simulink model "main_vehicle_v2"  (R2024b)
settings: Solver=FixedStepAuto  StartTime=0.0  StopTime=5  FixedStep=Ts  MaxStep=0.001  RelTol=1e-3
values from neighbouring files (symbols this model uses):
  Frr = Crr*m*g    (= 51.993)    [main_data_vehicle.m]    (also in xopt_launch.mat)
  lf = L*fr    (= 0.7905)    [main_data_vehicle.m]    (also in xopt_launch.mat)
  Re = 0.235    [main_data_vehicle.m]    (also in xopt_launch.mat)
  t_vec = (0:dt:simTime)'    [buildControlProfile.m]    (also in buildControlProfile2.m; optimal_launch_pedal_goodyear.mat = [0 0.001 0.002 0.003 0.004 0.005 0.006 0.007 0.008 0.009 0.0; optimal_launch_pedal_refined.mat = [0 0.001 0.002 0.003 0.004 0.005 0.006 0.007 0.008 0.009 0.0; optimal_launch_pedal_result.mat = [0 0.001 0.002 0.003 0.004 0.005 0.006 0.007 0.008 0.009 0.0)
  TirePressure = 65e3    (= 65000)    [main_data_vehicle.m]    (also in xopt_launch.mat)
  Ts = 0.001    [main_data_vehicle.m]    (also in xopt_launch.mat)
  u_vec = min(max(u_vec, uMin), uMax)    [buildControlProfile.m]    (also in buildControlProfile2.m; optimal_launch_pedal_goodyear.mat = [0.4076171875 0.409837690443 0.412058165147 0.414278583859 0; optimal_launch_pedal_refined.mat = [0.90859375 0.907017815717 0.905446650732 0.903880250909 0.9; optimal_launch_pedal_result.mat = [0.2 0.202202584529 0.204404077869 0.206604464652 0.20880372)
  v0 = 0    [main_data_vehicle.m]    (also in xopt_launch.mat)
undefined symbols (not defined in the file or in its folder): Sim3dSensor
libraries: simulink x3, sim3dlib x3, sim3dautolib x1, dspvision x1
settings Model: Creator=marti  LastModifiedBy=marti

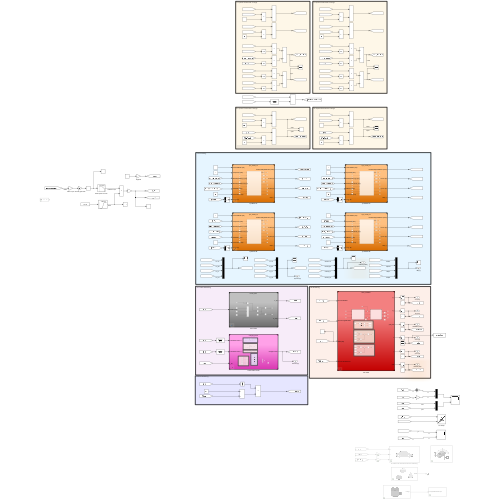
[thumbnail: Simulink's stored preview of the top-level diagram]
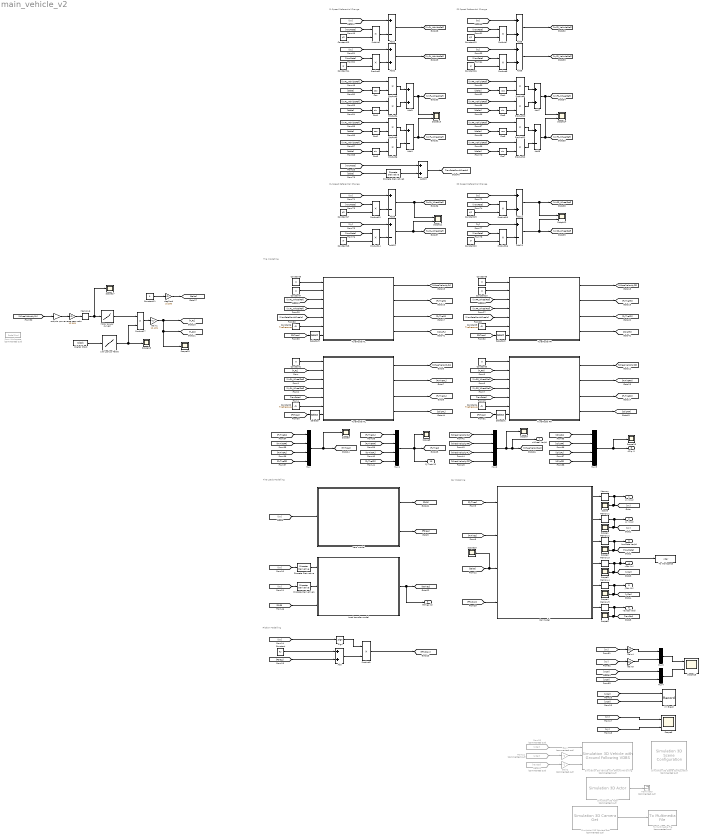
== system main_vehicle_v2 ==
  note: FL Speed Referential Change
  note: Car Modelling
  note: Friction Modelling
  note: Tire Loads Modelling
  note: Tire modelling
  note: FR Speed Referential Change
  note: RL Speed Referential Change
  note: RR Speed Referential Change
  1-D Lookup Table : Lookup_n-D  NumberOfTableDimensions=1  BreakpointsForDimension1=t_vec  Table=u_vec  InternalRulePriority=Speed  RndMeth=Simplest
  Add{,2..3,5..7,12..13} (8 alike) : Sum
  Add{1,4,8..11} (6 alike) : Sum  Inputs=+-
  Aero model : ModelReference  ModelNameDialog=forces_aero.slx  SimulationMode=Normal  ModelReferenceVersion=1.8
  Car model : ModelReference  ModelNameDialog=state_variables.slx  SimulationMode=Normal  ModelReferenceVersion=1.15
  Constant : Constant  Value=Frr
  Constant{1,3,5,7..8,10..11} (7 alike) : Constant  Value=0
  Constant{13,15,17,19} (4 alike) : Constant  Value=t/2
  Constant{14,16,18,20} (4 alike) : Constant  Value=lf
  Constant{2,4,6,9} (4 alike) : Constant  Value=TirePressure
  Cos{,2,4,6} (4 alike) : Trigonometry  Operator=cos
  Cos{1,3,5,7} (4 alike) : Trigonometry
  Digital Clock : DigitalClock  SampleTime=Ts
  Discrete Derivative : simulink/Discrete/Discrete Derivative  gainval=1.0  ICPrevScaledInput=0.0  OutMin=[]  OutMax=[]  OutDataType=fixdt(1, 16)  OutScaling=2^-10  DoSatur=off
  Discrete Derivative1 : simulink/Discrete/Discrete Derivative  gainval=1.0  ICPrevScaledInput=0.0  OutMin=[]  OutMax=[]  OutDataType=fixdt(1, 16)  OutScaling=2^-10  DoSatur=off
  Discrete Derivative2 : simulink/Discrete/Discrete Derivative  gainval=1.0  ICPrevScaledInput=0.0  OutMin=[]  OutMax=[]  OutDataType=fixdt(1, 16)  OutScaling=2^-10  DoSatur=off
  From Workspace : FromWorkspace  Commented=on  VariableName=PedalCmd
  From20 : From  Commented=on  GotoTag=xCar
  From21 : From  Commented=on  GotoTag=yCar
  From22 : From  Commented=on  GotoTag=YawCar
  Gain : Gain  Commented=on  Gain=-1
  Gain1 : Gain  Gain=12.481
  Gain2 : Gain  Commented=on  Gain=-1
  Gain4 : Gain  Gain=3.6
  Gain5 : Gain  Gain=3.6
  Load transfer model : ModelReference  ModelNameDialog=charges_pneus.slx  SimulationMode=Normal  ModelReferenceVersion=1.26
  Memory : Memory  InitialCondition=v0
  Memory{1..5} (5 alike) : Memory
  Memory6 : Memory  InitialCondition=v0/Re
  Motor power curve2 : Lookup_n-D  NumberOfTableDimensions=1  BreakpointsForDimension1=[0 11500 20000 20001]  Table=[32 32 18 0]  ExtrapMethod=Clip  UseLastTableValue=on  InternalRulePriority=Speed  RndMeth=Simplest
  Mux{,1..2,5} (4 alike) : Mux
  Mux3 : Mux  Inputs=2
  Mux4 : Mux  Inputs=2
  Product{,1..17} (18 alike) : Product
  Scope{,1..5,7..10,16..19} (14 alike) : Scope
  Scope{6,11..15} (6 alike) : Scope  NumInputPorts=2
  Selector : Selector  InputPortWidth=4  IndexOptions=Index vector (dialog)  Indices=1  OutputSizes=1
  Selector1 : Selector  InputPortWidth=4  IndexOptions=Index vector (dialog)  Indices=2  OutputSizes=1
  Selector2 : Selector  InputPortWidth=4  IndexOptions=Index vector (dialog)  Indices=4  OutputSizes=1
  Selector3 : Selector  InputPortWidth=4  IndexOptions=Index vector (dialog)  Indices=3  OutputSizes=1
  Sign : Signum
  Simulation 3D Actor : sim3dlib/Simulation 3D Actor  Commented=on  ActorName=Sim3dActor5  ParentName=Scene Origin  Operation=Create at setup  InitScriptText=skidpadConePlacement  SampleTime=.03  Translation=single([0 0 0])  Rotation=single([0 0 0])  Scale=single([1 1 1])  aMode=5  ActorTag=Sim3dActor5  ActorType=Sim3dActor  ID=5
      settings: LibrarySourceBlock=sl3dlib/Simulation 3D/Simulation 3D Actor
  Simulation 3D Camera Get : sim3dlib/Simulation 3D Camera Get  Priority=1  Commented=on  sensorTag=Sim3dSensor�  sensorId=2  sensorName=Sim3dSensor�  vehTagList={'Scene Origin';'Sim3dActor1';'Sim3dActor2';'Sim3dActor3';'Sim3dActor4';'Sim3dActor5';'SimulinkVehicle1'}  vehTag=SimulinkVehicle1  mountLoc=Origin  offsetFlag=on  tmountOffset=[-8, 0, 1]  rmountOffset=[0, 0, 0]  HorizontalResolution=1280  VerticalResolution=720  HorizontalFOV=60  SampleTime=0.03  mountPoint=[-8 0 1]  mountOrientation=[0 0 0]  aMode=5  ID=2
      settings: LibrarySourceBlock=sl3dlib/Simulation 3D/Utilities/Simulation 3D Camera Get
  Simulation 3D Scene Configuration : sim3dlib/Simulation 3D Scene Configuration  Priority=0  Commented=on  ProjectFormat=Default Scenes  SceneDesc=Straight road  ProjectName=C:\Program Files\MATLAB\R2024b\toolbox\shared\sim3d_projects\automotive_project_windows\UE\WindowsNoEditor\VehicleSimulation.exe  ScenePath=/Game/Maps/HwStrght  EnableOpenDRIVE=off  vehTagList={'Custom';'Scene Origin';'Sim3dActor1';'Sim3dActor2';'Sim3dActor3';'Sim3dActor4';'Sim3dActor5';'SimulinkVehicle1'}  vehTag=SimulinkVehicle1  FreeCameraInitialTranslation=[0, 0, 0]  FreeCameraDefaultInitialTranslation=[-6, 0, 2]  FreeCameraInitialRotation=[0, 0, 0]  FreeCameraDefaultInitialRotation=[0, -15, 0]  OpVisEn=off  Ts=.03  EnableWindow=on  EnableRemoteAccess=off  EnableWeather=off  SunAzimuth=90  SunAltitude=40.0  EnableGeospatialSun=off  Latitude=0  Longitude=0  Date=2023-01-01  Time=10:30:00  GeoTimeZone=-5.0  SunDaylightSaving=off  wind=1  clouds=10  EnableVolumetricClouds=off  CloudCoverage=0  CloudAltitude=6  fog=0  rain=0  RaindropsEffect=off  SnowDensity=0  EnableGeospatial=off  UseTrueOrigin=off  OriginHeight=200  OriginLatitude=40.744652  OriginLongitude=-73.988864  MapStyle=Aerial  AdditionalAssetIDs=[]  UseAdvancedSunSky=off  SolarTime=11  TimeZone=-5  Day=21  Month=9  Year=2022  UseDaylightSavingTime=on  DSTStartDay=10  DSTStartMonth=3  DSTEndDay=3  DSTEndMonth=11  DSTSwitchHour=2  sensorTag=MainCamera1  sensorId=1  sensorName=MainCamera1  mountLoc=Origin  offsetFlag=off  tmountOffset=[0, 0, 0]  rmountOffset=[0, 0, 0]  HorizontalResolution=1280  VerticalResolution=720  HorizontalFOV=60  mountPoint=[0 0 0]  mountOrientation=[0 0 0]  aMode=2  ID=1  GeoTrigger=Inactive
      settings: LibrarySourceBlock=vehdynlibsim3dcore/Simulation 3D Scene Configuration
  Simulation 3D Vehicle with Ground Following : sim3dautolib/Simulation 3D Vehicle with Ground Following VDBS  Priority=-1  Commented=on  PassVehMesh=Formula student vehicle  MeshPath=/MathWorksAutomotiveContent/Vehicles/Muscle/Meshes/SK_MuscleCar.SK_MuscleCar  TrackWidth=1.9  WheelBase=3  WheelRadius=0.35  VehColor=Silver  InitialPos=[0, 0, 0]  InitialRot=[0, 0, 0]  ActorName=SimulinkVehicle1  VehLightsControl=off  HeadlightColor=[ 1, 1, 1 ]  HighBeamIntensity=100000  LowBeamIntensity=60000  HighBeamConeAngle=1.22  LowBeamConeAngle=1.22  LeftHeadlightOrientation=[ 0, 0 ]  RightHeadlightOrientation=[ 0, 0 ]  BrakelightIntensity=200  ReverselightIntensity=500  SignallightIntensity=500  SignallightPeriod=1  SignalPulseWidth=50  SampleTime=-1  ActorType=SimulinkVehicle  ID=1  aMode=2  ActorTag=SimulinkVehicle1  CoordinateScheme=SAE
      settings: LibrarySourceBlock=vehdynlibsim3d/Simulation 3D Vehicle with Ground Following
  Terminator : Terminator  Commented=on
  To Multimedia File : dspvision/To Multimedia File  Commented=on  outputFilename=C:\Users\marti\Documents\EPSA\Travaux torque structure\SKIDPAD.mp4  streamSelection=Video only  videoCompressor=None (uncompressed)  audioCompressor=None (uncompressed)  imagePorts=One multidimensional signal  fileType=MPEG4  audioDatatype=Determine from input data type  fourcc=RGB  audioBitRate=128  audioQuality=75  videoQuality=75  mj2000CompFactor=10
      settings: LibrarySourceBlock=visionsinks/To Multimedia File
  To Workspace : ToWorkspace  VariableName=xCar  SaveFormat=Timeseries  SampleTime=Ts
  TyreModel FL : ModelReference  ModelNameDialog=tyre_model_v3.slx  SimulationMode=Normal  ModelReferenceVersion=1.26
  TyreModel FR : ModelReference  ModelNameDialog=tyre_model_v3.slx  SimulationMode=Normal  ModelReferenceVersion=1.26
  TyreModel RL : ModelReference  ModelNameDialog=tyre_model_v3.slx  SimulationMode=Normal  ModelReferenceVersion=1.26
  TyreModel RR : ModelReference  ModelNameDialog=tyre_model_v3.slx  SimulationMode=Normal  ModelReferenceVersion=1.26
  XY Graph : Record  FileSettingsInternal="{\"entries\":[{\"content\":{\"excelSettings\":{\"content\":{},\"type\":\"Streamout.ExcelSettings\"}},\"type\":\"Streamout.FileSettingStorage\",\"uuid\":\"\"}],\"packageUris\":[\"http:\\/\\/schema.mathworks.com\\/mf0\\/streamout_blocks\\/R2020a\"],\"version\":\"1.0\"}"  Layout=[1 1]  SignalsInternal="{\"entries\":[{\"content\":{\"signals\":[{\"content\":{\"blockPath\":[],\"dimensions\":[1],\"domain\":\"\",\"lineColor\":\"#0072bd\",\"lineWidth\":2,\"plots\":[ 1 ],\"port\":1,\"sid\":[\"\"],\"signalID\":1,\"signalName\":\"From16\"},\"type\":\"RecordBlkView.Signal\",\"uuid\":\"\"},{\"content\":{\"blockPath\":[],\"dimensions\":[1],\"domain\":\"\",\"lineColor\":\"#d95319\",\"lineWidth\":2,\"plots\":[ 1 ],\"port\":2,\"sid\":[\"\"],\"signalID\":2,\"signalName\":\"From15\"},\"type\":\"RecordBlkView.Signal\",\"uuid\":\"\"}]},\"type\":\"RecordBlkView.InputSignals\",\"uuid\":\"\"}],\"packageUris\":[\"http:\\/\\/schema.mathworks.com\\/mf0\\/streamout_blocks\\/R2020a\"],\"version\":\"1.0\"}"  VisualizationBindings="{\"xyplotplugin\":{\"info\":[{\"series\":[{\"bindingParametersList\":[{\"parameter\":\"X-Axis\",\"signalID\":1,\"signalName\":\"From16\"},{\"parameter\":\"Y-Axis\",\"signalID\":2,\"signalName\":\"From15\"}],\"seriesID\":0}],\"subplotID\":1}]}}"  CompatibilityTag=XY
  deg2rad : Gain  Gain=pi/180
  rad/s to rpm : Gain  Gain=30/pi
  reverse gear ratio : Gain  Gain=12.481
  Vx (m/s) : Outport
  Vy (m/s) : Outport  Port=2
  YawRate (rad/s) : Outport  Port=3
  xCar (m) : Outport  Port=4
  yCar (m) : Outport  Port=5
  YawCar (rad) : Outport  Port=6
  nWheel (rad/s) : Outport  Port=7
  rSlip (-) : Outport  Port=8
  FzTires (N) : Outport  Port=9
  FyTires (N) : Outport  Port=10
  wires:
  Car model/1 -> Memory/1
  Car model/2 -> Memory1/1
  Car model/3 -> Memory2/1
  Car model/4 -> Memory3/1
  Car model/5 -> Memory4/1
  Car model/6 -> Memory5/1
  [Vx] -> Aero model/1
  Memory/1 -> Vx (m/s)/1, Scope/1, [Vx]
  Memory1/1 -> Vy (m/s)/1, Scope1/1, [Vy]
  Memory2/1 -> YawRate (rad/s)/1, [YawRate], Scope2/1
  Memory3/1 -> To Workspace/1, xCar (m)/1, Scope3/1, [xCar]
  Memory4/1 -> yCar (m)/1, [yCar], Scope4/1
  Memory5/1 -> YawCar (rad)/1, Scope5/1, [YawCar]
  [Vx] -> Discrete Derivative/1
  Discrete Derivative/1 -> Load transfer model/1
  [Vy] -> Discrete Derivative1/1
  Discrete Derivative1/1 -> Load transfer model/2
  [FxTires] -> Car model/2
  [FyTires] -> Car model/1
  [delta] -> Scope10/1, Car model/3
  Aero model/2 -> [FDrag]
  [FDrag] -> Add/2
  Constant/1 -> Add/1
  [FFriction] -> Car model/4
  Add/1 -> Product1/2
  Load transfer model/1 -> FzTires (N)/1, [FzTires]
  [Vx] -> Sign/1
  Sign/1 -> Product1/1
  [yCar] -> XY Graph/2
  [xCar] -> XY Graph/1
  [Vx] -> Scope6/1  "v_x"
  [Vy] -> Scope6/2  "v_y"
  From20/1 -> Simulation 3D Vehicle with Ground Following/1
  From21/1 -> Gain/1
  From22/1 -> Gain2/1
  Gain/1 -> Simulation 3D Vehicle with Ground Following/2
  Gain2/1 -> Simulation 3D Vehicle with Ground Following/3
  Simulation 3D Actor/1 -> Terminator/1
  Simulation 3D Camera Get/1 -> To Multimedia File/1
  Constant1/1 -> TyreModel RL/1
  [T_RL] -> TyreModel RL/2
  [VxRL_WheelRef] -> TyreModel RL/3
  [VyRL_WheelRef] -> TyreModel RL/4
  [YawRate] -> TyreModel RL/5
  Constant2/1 -> TyreModel RL/6
  TyreModel RL/1 -> [WheelVelocityRL]
  TyreModel RL/2 -> [FxTireRL]
  TyreModel RL/3 -> [FyTireRL]
  TyreModel RR/3 -> [FyTireRR]
  TyreModel RR/2 -> [FxTireRR]
  TyreModel RR/1 -> [WheelVelocityRR]
  Constant4/1 -> TyreModel RR/6
  [YawRate] -> TyreModel RR/5
  [VyRR_WheelRef] -> TyreModel RR/4
  [VxRR_WheelRef] -> TyreModel RR/3
  [T_RR] -> TyreModel RR/2
  Constant3/1 -> TyreModel RR/1
  TyreModel FL/3 -> [FyTireFL]
  TyreModel FL/2 -> [FxTireFL]
  TyreModel FL/1 -> [WheelVelocityFL]
  Constant6/1 -> TyreModel FL/6
  [YawRateFrontWheels] -> TyreModel FL/5
  [VyFL_WheelRef] -> TyreModel FL/4
  [VxFL_WheelRef] -> TyreModel FL/3
  Constant7/1 -> TyreModel FL/2
  Constant5/1 -> TyreModel FL/1
  Constant8/1 -> TyreModel FR/1
  Constant10/1 -> TyreModel FR/2
  [VxFR_WheelRef] -> TyreModel FR/3
  [VyFR_WheelRef] -> TyreModel FR/4
  [YawRateFrontWheels] -> TyreModel FR/5
  Constant9/1 -> TyreModel FR/6
  TyreModel FR/1 -> [WheelVelocityFR]
  TyreModel FR/2 -> [FxTireFR]
  TyreModel FR/3 -> [FyTireFR]
  Aero model/1 -> [FLift]
  Product1/1 -> [FFriction]
  [FzTires] -> Selector/1
  Selector/1 -> TyreModel RL/7
  [FzTires] -> Selector1/1
  Selector1/1 -> TyreModel RR/7
  [FzTires] -> Selector2/1
  Selector2/1 -> TyreModel FR/7
  [FzTires] -> Selector3/1
  Selector3/1 -> TyreModel FL/7
  [FxTireRL] -> Mux/1  "Fx_RL"
  [FxTireRR] -> Mux/2  "Fx_RR"
  [FxTireFL] -> Mux/3  "Fx_FL"
  [FxTireFR] -> Mux/4  "Fx_FR"
  Mux/1 -> Scope9/1, [FxTires]
  Mux1/1 -> FyTires (N)/1, Scope8/1, [FyTires]
  [FyTireFR] -> Mux1/4  "Fy_FR"
  [FyTireFL] -> Mux1/3  "Fy_FL"
  [FyTireRR] -> Mux1/2  "Fy_RR"
  [FyTireRL] -> Mux1/1  "Fy_RL"
  Mux2/1 -> Scope7/1, nWheel (rad/s)/1, [WheelVelocities]
  [WheelVelocityRL] -> Mux2/1  "nWheel_RL"
  [WheelVelocityRR] -> Mux2/2  "nWheel_RR"
  [WheelVelocityFL] -> Mux2/3  "nWheel_FL"
  [WheelVelocityFR] -> Mux2/4  "nWheel_FR"
  [FLift] -> Load transfer model/3
  [Vx] -> Add1/1
  Product/1 -> Add1/2
  [YawRate] -> Product/1
  Constant13/1 -> Product/2
  Add1/1 -> [VxFL_VehicleRef]
  Add2/1 -> [VyFL_VehicleRef]
  Constant14/1 -> Product2/2
  [YawRate] -> Product2/1
  Product2/1 -> Add2/2
  [Vy] -> Add2/1
  [delta] -> Cos/1
  Cos/1 -> Product3/2
  [VxFL_VehicleRef] -> Product3/1
  [VyFL_VehicleRef] -> Product4/1
  Cos1/1 -> Product4/2
  [delta] -> Cos1/1
  Product3/1 -> Add3/1
  Product4/1 -> Add3/2
  Add3/1 -> Scope13/1, [VxFL_WheelRef]  "VxFL"
  Add4/1 -> Scope13/2, [VyFL_WheelRef]  "VyFL"
  Product6/1 -> Add4/2
  Product5/1 -> Add4/1
  [delta] -> Cos3/1
  Cos3/1 -> Product6/2
  [VxFL_VehicleRef] -> Product6/1
  [VyFL_VehicleRef] -> Product5/1
  Cos2/1 -> Product5/2
  [delta] -> Cos2/1
  [delta] -> Cos6/1
  Cos6/1 -> Product11/2
  [VyFR_VehicleRef] -> Product11/1
  [VxFR_VehicleRef] -> Product12/1
  Cos7/1 -> Product12/2
  [delta] -> Cos7/1
  Product11/1 -> Add8/1
  Product12/1 -> Add8/2
  Add8/1 -> Scope14/2, [VyFR_WheelRef]  "VyFR"
  Product10/1 -> Add7/2
  Product9/1 -> Add7/1
  [delta] -> Cos5/1
  Cos5/1 -> Product10/2
  [VyFR_VehicleRef] -> Product10/1
  [VxFR_VehicleRef] -> Product9/1
  Cos4/1 -> Product9/2
  [delta] -> Cos4/1
  [Vy] -> Add6/1
  Product8/1 -> Add6/2
  [YawRate] -> Product8/1
  Constant16/1 -> Product8/2
  Add6/1 -> [VyFR_VehicleRef]
  Add5/1 -> [VxFR_VehicleRef]
  Constant15/1 -> Product7/2
  [YawRate] -> Product7/1
  Product7/1 -> Add5/2
  [Vx] -> Add5/1
  [Vy] -> Add10/1
  Product14/1 -> Add10/2
  [YawRate] -> Product14/1
  Constant18/1 -> Product14/2
  Add10/1 -> Scope11/2, [VyRL_WheelRef]  "VyRL"
  Add9/1 -> Scope11/1, [VxRL_WheelRef]  "VxRL"
  Constant17/1 -> Product13/2
  [YawRate] -> Product13/1
  Product13/1 -> Add9/2
  [Vx] -> Add9/1
  [Vx] -> Add12/1
  Product15/1 -> Add12/2
  [YawRate] -> Product15/1
  Constant19/1 -> Product15/2
  Add12/1 -> Scope12/1, [VxRR_WheelRef]  "VxRR"
  Add11/1 -> Scope12/2, [VyRR_WheelRef]  "VyRR"
  Constant20/1 -> Product16/2
  [YawRate] -> Product16/1
  Product16/1 -> Add11/2
  [Vy] -> Add11/1
  Discrete Derivative2/1 -> Add13/2
  [YawRate] -> Add13/1
  Add13/1 -> [YawRateFrontWheels]
  [delta] -> Discrete Derivative2/1
  Add7/1 -> Scope14/1, [VxFR_WheelRef]  "VxFR"
  Product17/1 -> Gain1/1
  Constant11/1 -> deg2rad/1
  Mux5/1 -> Scope16/1, rSlip (-)/1
  Gain5/1 -> Mux3/2  "v_y"
  Gain4/1 -> Mux3/1  "v_x"
  [Vy] -> Gain5/1  "v_y"
  [Vx] -> Gain4/1  "v_x"
  Mux3/1 -> Scope15/1
  [xCar] -> Mux4/1  "xCar"
  [yCar] -> Mux4/2  "yCar"
  Mux4/1 -> Scope15/2
  deg2rad/1 -> [delta]
  TyreModel FL/4 -> [rSlipFL]
  TyreModel FR/4 -> [rSlipFR]
  TyreModel RR/4 -> [rSlipRR]
  TyreModel RL/4 -> [rSlipRL]
  [rSlipFR] -> Mux5/4  "rSlipFR"
  [rSlipFL] -> Mux5/3  "rSlipFL"
  [rSlipRR] -> Mux5/2  "rSlipRR"
  [rSlipRL] -> Mux5/1  "rSlipRL"
  Motor power curve2/1 -> Product17/1  "available torque"
  [WheelVelocityRL] -> rad/s to rpm/1  "nMotor"
  Memory6/1 -> Scope17/1, Motor power curve2/1
  Gain1/1 -> Scope19/1, [T_RR], [T_RL]
  rad/s to rpm/1 -> reverse gear ratio/1
  reverse gear ratio/1 -> Memory6/1
  Digital Clock/1 -> 1-D Lookup Table/1
  1-D Lookup Table/1 -> Scope18/1, Product17/2  "APPS"
